simulink model "VEKF"  (R2018a)
settings: Solver=VariableStepAuto  StartTime=0.0  StopTime=10.0  RelTol=1e-3
PreLoadFcn:
  | modelDir = fileparts(get_param(bdroot, 'FileName'));
  | addpath(fullfile(modelDir,'../../Parameters'));
  | addpath(fullfile(modelDir,'../../Estimators/VEKF'));
  | 
  | Parameters_Estimators
  | Parameters_Simulation
InitFcn:
  | Parameters_Estimators
  | Parameters_Simulation
undefined symbols (not defined in the file or in its folder): constants_nominal, cov_acc, eta_accelerometer, eta_encoder, TicksPrRev, Ts, var_acc_bias, var_acceleration, VelocityEstimator_P_init_diagonal
libraries: simulink x1
settings Model: Creator=Thomas  LastModifiedBy=Thomas

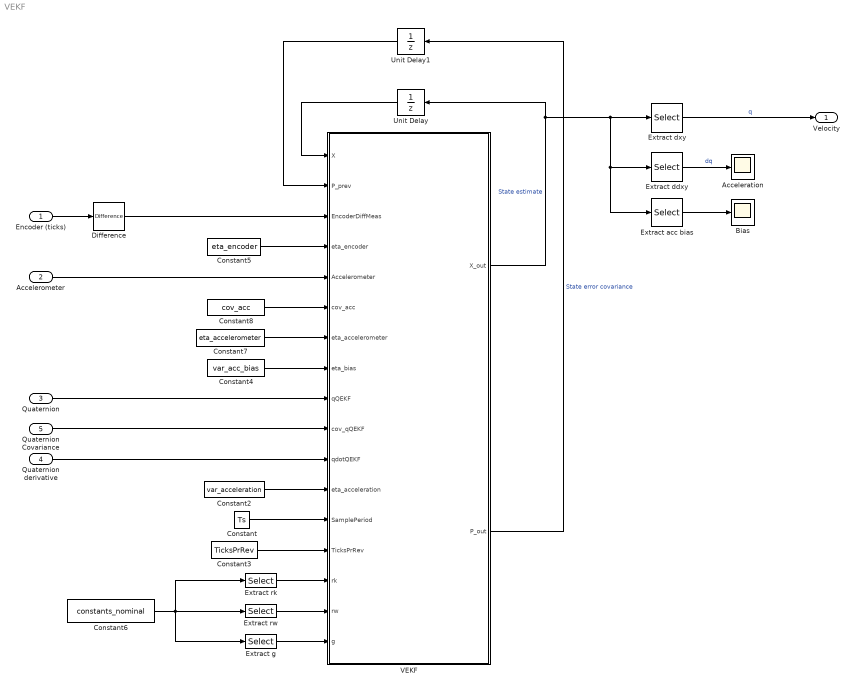
== system VEKF ==
  Encoder (ticks) : Inport  PortDimensions=3
  Accelerometer : Inport  Port=2
  Quaternion : Inport  Port=3
  Quaternion derivative : Inport  Port=4
  Quaternion Covariance : Inport  Port=5
  Acceleration : Scope
  Bias : Scope
  Constant : Constant  Value=Ts
  Constant2 : Constant  Value=var_acceleration
  Constant3 : Constant  Value=TicksPrRev
  Constant4 : Constant  Value=var_acc_bias
  Constant5 : Constant  Value=eta_encoder
  Constant6 : Constant  Value=constants_nominal
  Constant7 : Constant  Value=eta_accelerometer
  Constant8 : Constant  Value=cov_acc
  "Difference " : simulink/Discrete/Difference  ICPrevInput=0.0  OutMin=[]  OutMax=[]  OutDataType=fixdt(1, 16)  OutScaling=2^-10  DoSatur=off
  Extract acc bias : Selector  InputPortWidth=7  IndexOptions=Index vector (dialog)  Indices=[5 6 7]  OutputSizes=1
  Extract ddxy : Selector  InputPortWidth=7  IndexOptions=Index vector (dialog)  Indices=[3 4]  OutputSizes=1
  Extract dxy : Selector  InputPortWidth=7  IndexOptions=Index vector (dialog)  Indices=[1 2]  OutputSizes=1
  Extract g : Selector  InputPortWidth=13  IndexOptions=Index vector (dialog)  Indices=[13]  OutputSizes=1
  Extract rk : Selector  InputPortWidth=13  IndexOptions=Index vector (dialog)  Indices=[3]  OutputSizes=1
  Extract rw : Selector  InputPortWidth=13  IndexOptions=Index vector (dialog)  Indices=[9]  OutputSizes=1
  Unit Delay : UnitDelay  InitialCondition=zeros(7,1);  SampleTime=Ts
  Unit Delay1 : UnitDelay  InitialCondition=diag(VelocityEstimator_P_init_diagonal)  SampleTime=Ts
  VEKF : MATLAB Function  TreatAsAtomicUnit=on
  Velocity : Outport
  wires:
  Unit Delay1/1 -> VEKF/2(P_prev)
  Extract g/1 -> VEKF/17(g)
  VEKF/2(P_out) -> Unit Delay1/1  "State error covariance"
  VEKF/1(X_out) -> Unit Delay/1, Extract acc bias/1, Extract ddxy/1, Extract dxy/1  "State estimate"
  Extract acc bias/1 -> Bias/1
  Unit Delay/1 -> VEKF/1(X)
  Encoder (ticks)/1 -> "Difference "/1
  "Difference "/1 -> VEKF/3(EncoderDiffMeas)
  Constant/1 -> VEKF/13(SamplePeriod)
  Constant3/1 -> VEKF/14(TicksPrRev)
  Extract rw/1 -> VEKF/16(rw)
  Extract rk/1 -> VEKF/15(rk)
  Constant6/1 -> Extract g/1, Extract rw/1, Extract rk/1
  Constant2/1 -> VEKF/12(eta_acceleration)
  Constant5/1 -> VEKF/4(eta_encoder)
  Constant4/1 -> VEKF/8(eta_bias)
  Constant7/1 -> VEKF/7(eta_accelerometer)
  Constant8/1 -> VEKF/6(cov_acc)
  Accelerometer/1 -> VEKF/5(Accelerometer)
  Quaternion/1 -> VEKF/9(qQEKF)
  Quaternion derivative/1 -> VEKF/11(qdotQEKF)
  Quaternion Covariance/1 -> VEKF/10(cov_qQEKF)
  Extract ddxy/1 -> Acceleration/1  "dq"
  Extract dxy/1 -> Velocity/1  "q"

== matlab function VEKF/VEKF ==
  data: X input size=7; P_prev input size=[7,7]; X_out output size=7; EncoderDiffMeas input size=3; eta_encoder input size=1; Accelerometer input size=3; cov_acc input; eta_accelerometer input; eta_bias input; qQEKF input size=4; cov_qQEKF input size=[4,4]; qdotQEKF input size=4; eta_acceleration input; P_out output size=[7,7]; SamplePeriod input; TicksPrRev input; rk input; rw input; g input
function [X_out, P_out] = VelocityEKF_(X, P_prev, EncoderDiffMeas, eta_encoder, Accelerometer, cov_acc, eta_accelerometer, eta_bias, qQEKF, cov_qQEKF, qdotQEKF, eta_acceleration, SamplePeriod, TicksPrRev, rk,rw,g)
    [X_out_, P_out_] = VelocityEKF(single(X), single(P_prev), single(EncoderDiffMeas), single(eta_encoder), single(Accelerometer), single(cov_acc), single(eta_accelerometer), single(eta_bias), single(qQEKF), single(cov_qQEKF), single(qdotQEKF), single(eta_acceleration), single(SamplePeriod), single(TicksPrRev), single(rk), single(rw), single(g));
    X_out = double(X_out_);
    P_out = double(P_out_);
end
